simulink subsystem "Gesamtmodell"  (R2020a)
settings: Solver=VariableStepAuto  StartTime=0.0  StopTime=10.0  RelTol=1e-3
model mask{ModellParameter=0}
Description:
  | Gesamtmodell des Versuchsaufbaus
  | Eingang: Spannung
  | Ausgang: Pendelwinkel, alle Zustände
settings Model: Creator=Tobias  LastModifiedBy=Tobias

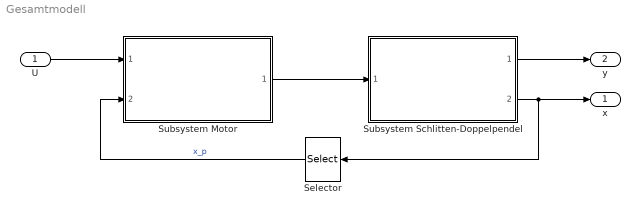
== system Gesamtmodell ==
  U : Inport
  Selector : Selector  InputPortWidth=6  IndexOptions=Index vector (dialog)  Indices=[2]  OutputSizes=1
  Subsystem Motor : Subsystem  ReferencedSubsystem=Motor  motorSimParams=ModellParameter.motor  K_UI=0  T_UI=0  K_I=0  J_MG=0  K_G=0  r32=0  d0_MG=0  dw_MG=0  Imax=0  Umax_out=0  Umax_in=0  R=0
  Subsystem Schlitten-Doppelpendel : Subsystem  ReferencedSubsystem=SchlittenPendel  params=ModellParameter.schlittenpendel
  x : Outport
  y : Outport  Port=2
  wires:
  Subsystem Motor/1 -> Subsystem Schlitten-Doppelpendel/1
  Subsystem Schlitten-Doppelpendel/1 -> y/1
  U/1 -> Subsystem Motor/1
  Subsystem Schlitten-Doppelpendel/2 -> Selector/1, x/1
  Selector/1 -> Subsystem Motor/2  "x_p"
